simulink model "PTC_MBDS_StringSource_Sample"  (R2013a)
settings: Solver=FixedStepDiscrete  StartTime=0.0  StopTime=100  FixedStep=0.02  RelTol=1e-3
libraries: PTC_MBDS_LIB x2, simulink_extras x1
settings Model: Creator=uidl7367  LastModifiedBy=sundeep.tuteja
settings DataIOCC: SignalLoggingSaveFormat=ModelDataLogs
settings OptimizationCC: ExpressionDepthLimit=2147483647  InitFltsAndDblsToZero=on
settings DebuggingCC: SaveWithParameterizedLinksMsg=none  SignalResolutionControl=TryResolveAllWithWarning  SolverPrmCheckMsg=none  InheritedTsInSrcMsg=none  MultiTaskDSMMsg=warning  MultiTaskCondExecSysMsg=none  FcnCallInpInsideContextMsg=UseLocalSettings  StrictBusMsg=Warning
settings RTWCC: IncludeERTFirstTime=on
settings GRTTargetCC: TargetFcnLib=ansi_tfl_tmw.mat  CombineOutputUpdateFcns=off  GRTInterface=on

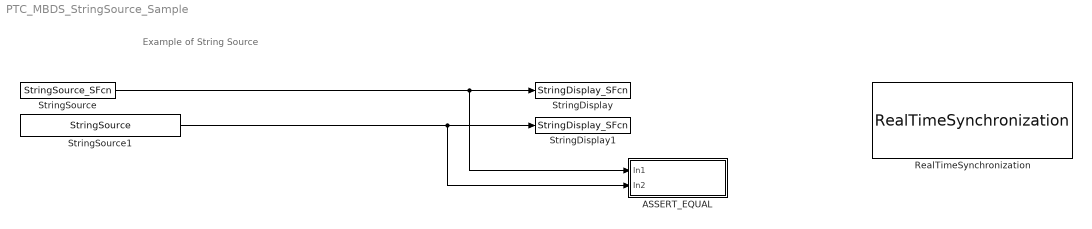
== system PTC_MBDS_StringSource_Sample ==
  note: Example of String Source
  ASSERT_EQUAL : Subsystem
  RealTimeSynchronization : PTC_MBDS_LIB/MBDS Standard Library/Extended Operations/HMI/RealTimeSynchronization  Enable=off  PTC_MBDS_BlockVersion=5.32  PTC_BlockType=PTC_MBDS_RealTimeSynchronization
  StringDisplay : M-S-Function  InitFcn=|  FunctionName=StringDisplay_SFcn  Parameters=MaxRowCount  mask(StringDisplay){MBDS_LibraryBlock=on, MaxRowCount=1, MBDS_BlockVersion=05.20}
      | if(exist('MBDS_BlockCallback', 'file'))
      |    MBDS_BlockCallback('Update', gcb);
      | end
      mask prompts: MBDS_LibraryBlock "MBDS Library Block"; MaxRowCount "Maximum number of rows displayed (min. 1):"; MBDS_BlockVersion "Block version:"
      mask help: The string display block shows an uint8 array as ASCII strings on the block mask.
      mask init:
      | MBDS_BlockCallback('Copy', gcb);
      mask Help: eval(['open([workdir(''Library_Dir:''),''\Blockset\Help\'',get_param(gcb,''MaskType''),''.html''])'])
      mask Callback MaxRowCount:
      | if(str2double(get_param(gcb, 'MaxRowCount')) < 1)
      |    set_param(gcb, 'MaxRowCount', '1');
      | end
      mask Display: text(0.05,0.5,'MyString','horizontalAlignment','left','verticalAlignment','middle')
  StringDisplay1 : M-S-Function  InitFcn=|  FunctionName=StringDisplay_SFcn  Parameters=MaxRowCount  mask(StringDisplay){MBDS_LibraryBlock=on, MaxRowCount=1, MBDS_BlockVersion=05.20}
      | if(exist('MBDS_BlockCallback', 'file'))
      |    MBDS_BlockCallback('Update', gcb);
      | end
      mask prompts: MBDS_LibraryBlock "MBDS Library Block"; MaxRowCount "Maximum number of rows displayed (min. 1):"; MBDS_BlockVersion "Block version:"
      mask help: The string display block shows an uint8 array as ASCII strings on the block mask.
      mask init:
      | MBDS_BlockCallback('Copy', gcb);
      mask Help: eval(['open([workdir(''Library_Dir:''),''\Blockset\Help\'',get_param(gcb,''MaskType''),''.html''])'])
      mask Callback MaxRowCount:
      | if(str2double(get_param(gcb, 'MaxRowCount')) < 1)
      |    set_param(gcb, 'MaxRowCount', '1');
      | end
      mask Display: text(0.05,0.5,'MyString','horizontalAlignment','left','verticalAlignment','middle')
  StringSource : S-Function  InitFcn=|  FunctionName=StringSource_SFcn  Parameters=uint8(String), uint16(MaxStringLength)  EnableBusSupport=off  mask(StringSource){MBDS_LibraryBlock=on, InputValue=MyString, MBDS_BlockVersion=05.40}
      | if(exist('MBDS_BlockCallback', 'file'))
      |    MBDS_BlockCallback('Update', gcb);
      | end
      mask prompts: MBDS_LibraryBlock "MBDS Library Block"; InputValue "Constant value:"; MBDS_BlockVersion "Block version:"
      mask help: This block outputs an uint8 array based on the ASCII codes of the string specified by the user.
      mask init:
      | MBDS_BlockCallback('Copy', gcb);
      | MaxStringLength = 1 + GetStringLen();
      | DispString = 'Error';
      | String = InputValue;
      | % Skip if string specifies a numeric expression or starts with '
      | if(isempty(str2num(String)) && String(1) ~= '''')
      |    try
      |       % Try to evaluate project constant 
      |       String = evalin('base', String);
      |    end   
      | end
      | if ~ischar(String) || size(String, 1) > 1
      | 	error('String must be a [1xn] array of type ''char'' with at least one character')
      | else
      |    % Limit to max. string length
      |    String = String(1:min(MaxStringLength, length(String)));
      | 	DispString = InputValue;
      | end
      mask Help: eval(['open([workdir(''Library_Dir:''),''\Blockset\Help\'',get_param(gcb,''MaskType''),''.html''])'])
      mask Display: text(0.05,0.5,DispString,'horizontalAlignment','left')
  StringSource1 : PTC_MBDS_LIB/MBDS Standard Library/Extended Operations/String Operations/StringSource  InputValue=MyString  PTC_MBDS_BlockVersion=5.32  PTC_BlockType=PTC_MBDS_StringSource  Value=uint8([77; 121; 83; 116; 114; 105; 110; 103; 0; 0; 0; 0; 0; 0; 0; 0; 0; 0; 0; 0; 0; 0; 0; 0; 0; 0; 0; 0; 0; 0; 0; 0; 0; 0; 0; 0; 0; 0; 0; 0; 0])  MaxStringLength=PTC_MBDS_MaxStringLength_Fcn
  wires:
  StringSource/1 -> ASSERT_EQUAL/1(In1), StringDisplay/1
  StringSource1/1 -> ASSERT_EQUAL/2(In2), StringDisplay1/1

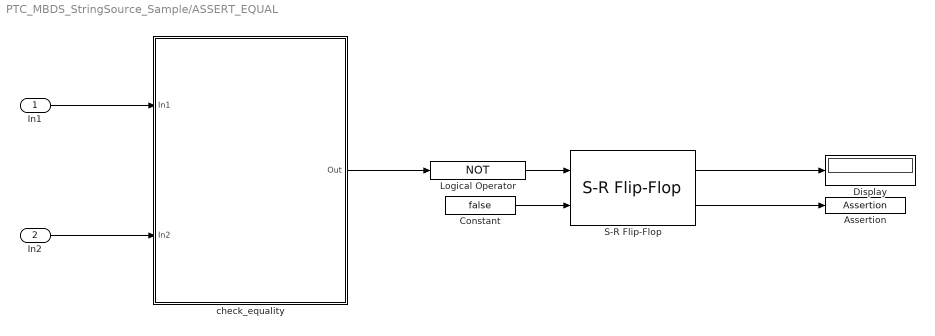
== system PTC_MBDS_StringSource_Sample/ASSERT_EQUAL ==
  In1 : Inport
  In2 : Inport  Port=2
  Assertion : Assertion
  Constant : Constant  Value=false
  Display : Display
  Logical Operator : Logic  Operator=NOT  AllPortsSameDT=off  OutDataTypeStr=boolean
  S-R Flip-Flop : simulink_extras/Flip Flops/S-R Flip-Flop  initial_condition=0
  check_equality : MATLAB Function  TreatAsAtomicUnit=on
  wires:
  S-R Flip-Flop/1 -> Display/1
  check_equality/1(Out) -> Logical Operator/1
  Constant/1 -> S-R Flip-Flop/2
  S-R Flip-Flop/2 -> Assertion/1
  In2/1 -> check_equality/2(In2)
  In1/1 -> check_equality/1(In1)
  Logical Operator/1 -> S-R Flip-Flop/1

== matlab function PTC_MBDS_StringSource_Sample/ASSERT_EQUAL/check_equality ==
  data: In1 input; Out output; In2 input
function Out = check_equality(In1, In2)
%#codegen

Out = isequaln(In1, In2);

end
